simulink model "plant_model_us06_ev_V06"  (R2018a)
settings: Solver=ode3  StartTime=0.0  StopTime=sim_time  FixedStep=0.01  RelTol=1e-3
values from neighbouring files (symbols this model uses):
  A = 2.0    (= 2)    [plant_model_us06_ev_V06_m.m]
  Cd = 0.3    [plant_model_us06_ev_V06_m.m]
  FDR = 10    [plant_model_us06_ev_V06_m.m]
  g = 9.81    [plant_model_us06_ev_V06_m.m]
  initial_speed = 0    [plant_model_us06_ev_V06_m.m]
  M = 2000    [plant_model_us06_ev_V06_m.m]
  max_torque = 400    [plant_model_us06_ev_V06_m.m]
  Mr = 0.015    [plant_model_us06_ev_V06_m.m]
  p = 1.225    [plant_model_us06_ev_V06_m.m]
  power_kW = 100    [plant_model_us06_ev_V06_m.m]
  r = 0.35    [plant_model_us06_ev_V06_m.m]
  radiant_angle = 0    [plant_model_us06_ev_V06_m.m]
undefined symbols (not defined in the file or in its folder): magnitude
libraries: simulink x2
settings Model: Creator=satven  LastModifiedBy=satven

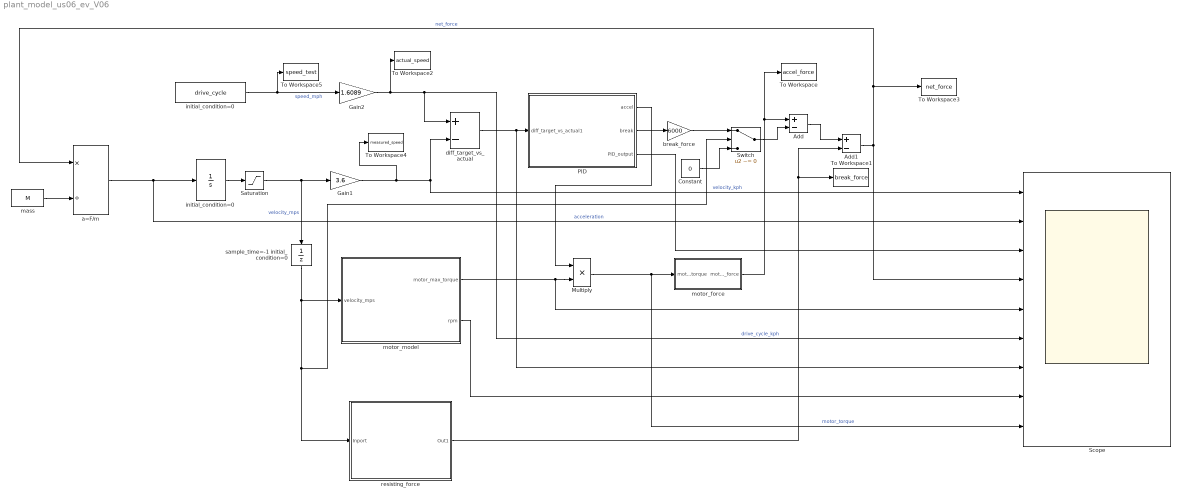
== system plant_model_us06_ev_V06 ==
  Add : Sum  Inputs=+-
  Add1 : Sum  Inputs=+-
  Constant : Constant  Value=0
  Gain1 : Gain  Gain=3.6
  Gain2 : Gain  Gain=1.6089
  Multiply : Product
  PID : Subsystem
  Saturation : Saturate  UpperLimit=inf  LowerLimit=0
  Scope : Scope  NumInputPorts=9
  Switch : Switch  Criteria=u2 ~= 0
  To Workspace : ToWorkspace  VariableName=accel_force  SaveFormat=Timeseries  SampleTime=-1
  To Workspace1 : ToWorkspace  VariableName=break_force  SaveFormat=Timeseries  SampleTime=-1
  To Workspace2 : ToWorkspace  VariableName=actual_speed  SaveFormat=Timeseries  SampleTime=-1
  To Workspace3 : ToWorkspace  VariableName=net_force  SaveFormat=Timeseries  SampleTime=-1
  To Workspace4 : ToWorkspace  VariableName=measured_speed  SaveFormat=Timeseries  SampleTime=-1
  To Workspace5 : ToWorkspace  VariableName=speed_test  SaveFormat=Timeseries  SampleTime=-1
  a=F/m : Product  Inputs=*/
  break_force : Gain  Gain=6000
  diff_target_vs_actual : Sum  Inputs=+-
  initial_condition=0 : Integrator  InitialCondition=initial_speed  LowerSaturationLimit=0
  "initial_condition=0 " : FromWorkspace  VariableName=drive_cycle  SampleTime=0.01
  mass : Constant  Value=M
  motor_force : Subsystem
  motor_model : Subsystem
  resisting_force : Subsystem
  "sample_time=-1 initial_condition=0 " : UnitDelay  SampleTime=-1
  wires:
  Gain1/1 -> To Workspace4/1, Scope/1, diff_target_vs_actual/2  "velocity_kph"
  diff_target_vs_actual/1 -> PID/1(diff_target_vs_actual1), Scope/7
  mass/1 -> a=F/m/2
  "sample_time=-1 initial_condition=0 "/1 -> motor_model/1(velocity_mps), Switch/2, resisting_force/1(Inport)
  a=F/m/1 -> initial_condition=0/1, Scope/2  "acceleration"
  Saturation/1 -> Gain1/1, "sample_time=-1 initial_condition=0 "/1  "velocity_mps"
  "initial_condition=0 "/1 -> Gain2/1, To Workspace5/1  "speed_mph"
  initial_condition=0/1 -> Saturation/1
  PID/3(PID_output) -> Scope/3
  Gain2/1 -> To Workspace2/1, diff_target_vs_actual/1, Scope/6  "drive_cycle_kph"
  Add/1 -> Add1/1
  PID/2(break) -> break_force/1
  motor_model/1(motor_max_torque) -> Scope/5, Multiply/2
  Add1/1 -> a=F/m/1, To Workspace3/1, Scope/4  "net_force"
  motor_model/2(rpm) -> Scope/8
  Multiply/1 -> Scope/9, motor_force/1(motor_torque)  "motor_torque"
  PID/1(accel) -> Multiply/1
  motor_force/1(motor_force) -> Add/1, To Workspace/1
  break_force/1 -> Switch/1
  Constant/1 -> Switch/3
  Switch/1 -> Add/2
  resisting_force/1(Out1) -> To Workspace1/1, Add1/2

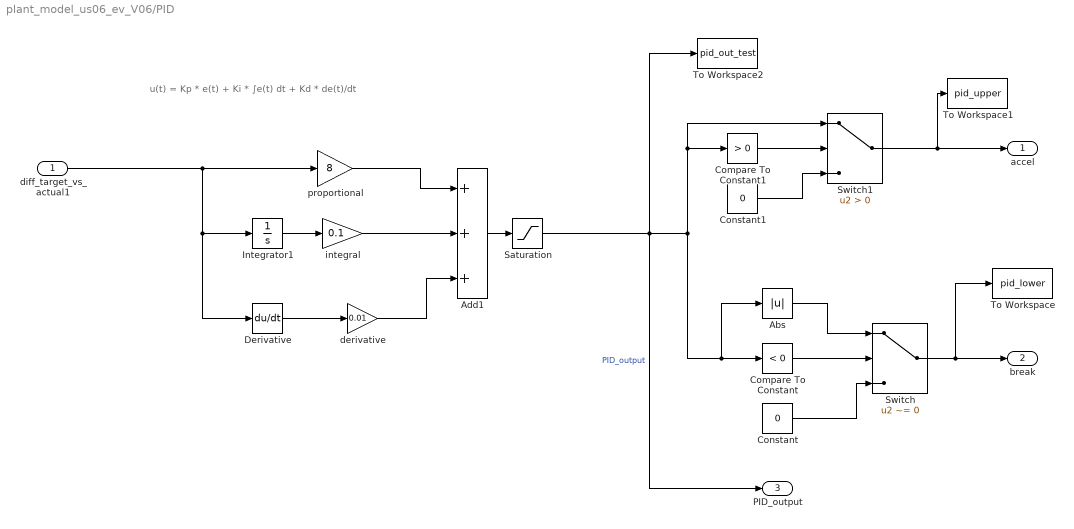
== system plant_model_us06_ev_V06/PID ==
  note: u(t) = Kp * e(t) + Ki * ∫e(t) dt + Kd * de(t)/dt
  diff_target_vs_actual1 : Inport
  Abs : Abs
  Add1 : Sum  Inputs=+++
  Compare To Constant : simulink/Logic and Bit Operations/Compare To Constant  relop=<  const=0  OutDataTypeStr=boolean
  Compare To Constant1 : simulink/Logic and Bit Operations/Compare To Constant  relop=>  const=0  OutDataTypeStr=boolean
  Constant : Constant  Value=0
  Constant1 : Constant  Value=0
  Derivative : Derivative
  Integrator1 : Integrator
  Saturation : Saturate  UpperLimit=1  LowerLimit=-1
  Switch : Switch  Criteria=u2 ~= 0
  Switch1 : Switch  Criteria=u2 > Threshold
  To Workspace : ToWorkspace  VariableName=pid_lower  SaveFormat=Timeseries  SampleTime=-1
  To Workspace1 : ToWorkspace  VariableName=pid_upper  SaveFormat=Timeseries  SampleTime=-1
  To Workspace2 : ToWorkspace  VariableName=pid_out_test  SaveFormat=Timeseries  SampleTime=-1
  "derivative " : Gain  Gain=0.01
  integral : Gain  Gain=0.1
  proportional : Gain  Gain=8
  accel : Outport
  break : Outport  Port=2
  PID_output : Outport  Port=3
  wires:
  proportional/1 -> Add1/1
  Derivative/1 -> "derivative "/1
  Integrator1/1 -> integral/1
  integral/1 -> Add1/2
  diff_target_vs_actual1/1 -> Derivative/1, Integrator1/1, proportional/1
  "derivative "/1 -> Add1/3
  Add1/1 -> Saturation/1
  Compare To Constant/1 -> Switch/2
  Compare To Constant1/1 -> Switch1/2
  Abs/1 -> Switch/1
  Constant/1 -> Switch/3
  Saturation/1 -> To Workspace2/1, PID_output/1, Abs/1, Compare To Constant/1, Switch1/1, Compare To Constant1/1  "PID_output"
  Switch/1 -> break/1, To Workspace/1
  Switch1/1 -> accel/1, To Workspace1/1
  Constant1/1 -> Switch1/3

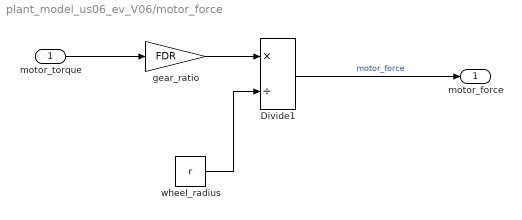
== system plant_model_us06_ev_V06/motor_force ==
  motor_torque : Inport
  Divide1 : Product  Inputs=*/
  gear_ratio : Gain  Gain=FDR
  wheel_radius : Constant  Value=r
  motor_force : Outport
  wires:
  motor_torque/1 -> gear_ratio/1
  wheel_radius/1 -> Divide1/2
  Divide1/1 -> motor_force/1  "motor_force"
  gear_ratio/1 -> Divide1/1

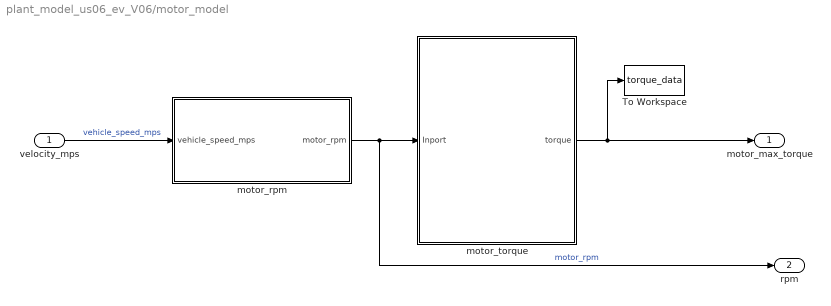
== system plant_model_us06_ev_V06/motor_model ==
  velocity_mps : Inport
  To Workspace : ToWorkspace  VariableName=torque_data  SaveFormat=Timeseries  SampleTime=-1
  motor_rpm : Subsystem
  motor_torque : Subsystem
  motor_max_torque : Outport
  rpm : Outport  Port=2
  wires:
  velocity_mps/1 -> motor_rpm/1(vehicle_speed_mps)  "vehicle_speed_mps"
  motor_torque/1(torque) -> To Workspace/1, motor_max_torque/1
  motor_rpm/1(motor_rpm) -> rpm/1, motor_torque/1(Inport)  "motor_rpm"

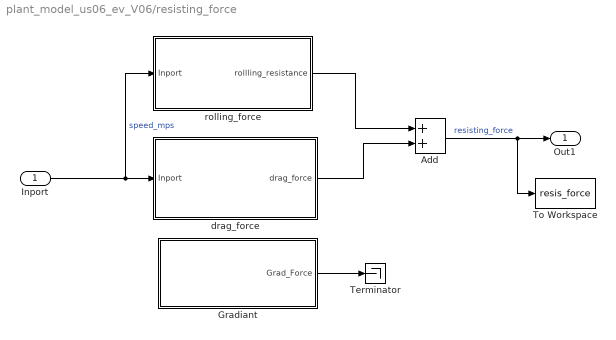
== system plant_model_us06_ev_V06/resisting_force ==
  Inport : Inport
  Add : Sum
  Gradiant : Subsystem
  Terminator : Terminator
  To Workspace : ToWorkspace  VariableName=resis_force  SaveFormat=Timeseries  SampleTime=-1
  drag_force : Subsystem
  rolling_force : Subsystem
  Out1 : Outport
  wires:
  drag_force/1(drag_force) -> Add/2
  Add/1 -> To Workspace/1, Out1/1  "resisting_force"
  rolling_force/1(rollling_resistance) -> Add/1
  Gradiant/1(Grad_Force) -> Terminator/1
  Inport/1 -> rolling_force/1(Inport), drag_force/1(Inport)  "speed_mps"

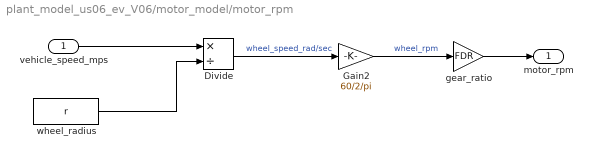
== system plant_model_us06_ev_V06/motor_model/motor_rpm ==
  vehicle_speed_mps : Inport
  Divide : Product  Inputs=*/
  Gain2 : Gain  Gain=60/2/pi
  gear_ratio : Gain  Gain=FDR
  wheel_radius : Constant  Value=r
  motor_rpm : Outport
  wires:
  wheel_radius/1 -> Divide/2
  Gain2/1 -> gear_ratio/1  "wheel_rpm"
  gear_ratio/1 -> motor_rpm/1
  Divide/1 -> Gain2/1  "wheel_speed_rad/sec"
  vehicle_speed_mps/1 -> Divide/1

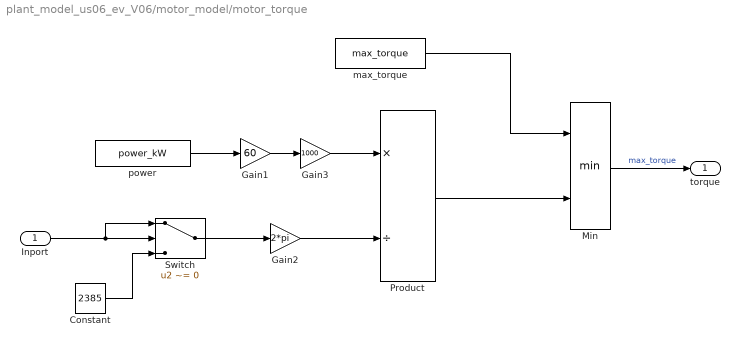
== system plant_model_us06_ev_V06/motor_model/motor_torque ==
  Inport : Inport
  Constant : Constant  Value=2385
  Gain1 : Gain  Gain=60
  Gain2 : Gain  Gain=2*pi
  Gain3 : Gain  Gain=1000
  Min : MinMax  Inputs=2
  Product : Product  Inputs=*/
  Switch : Switch  Criteria=u2 ~= 0
  max_torque : Constant  Value=max_torque
  power : Constant  Value=power_kW
  torque : Outport
  wires:
  power/1 -> Gain1/1
  Switch/1 -> Gain2/1
  Gain3/1 -> Product/1
  max_torque/1 -> Min/1
  Constant/1 -> Switch/3
  Gain2/1 -> Product/2
  Gain1/1 -> Gain3/1
  Product/1 -> Min/2
  Min/1 -> torque/1  "max_torque"
  Inport/1 -> Switch/1, Switch/2

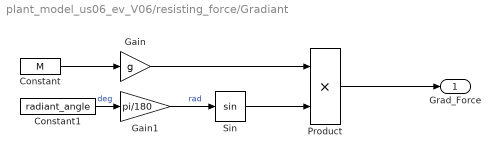
== system plant_model_us06_ev_V06/resisting_force/Gradiant ==
  Constant : Constant  Value=M
  Constant1 : Constant  Value=radiant_angle
  Gain : Gain  Gain=g
  Gain1 : Gain  Gain=pi/180
  Product : Product
  Sin : Trigonometry
  Grad_Force : Outport
  wires:
  Constant/1 -> Gain/1
  Product/1 -> Grad_Force/1
  Constant1/1 -> Gain1/1  "deg"
  Gain1/1 -> Sin/1  "rad"
  Gain/1 -> Product/1
  Sin/1 -> Product/2

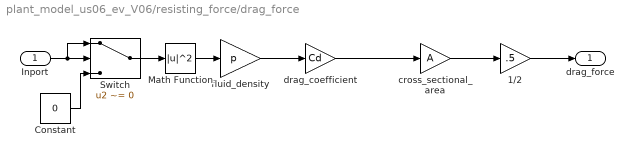
== system plant_model_us06_ev_V06/resisting_force/drag_force ==
  Inport : Inport
  1/2 : Gain  Gain=.5
  Constant : Constant  Value=0
  Math Function : Math  Operator=magnitude^2  OutputSignalType=real  SaturateOnIntegerOverflow=on
  Switch : Switch  Criteria=u2 ~= 0
  cross_sectional_area : Gain  Gain=A
  drag_coefficient : Gain  Gain=Cd
  fluid_density : Gain  Gain=p
  drag_force : Outport
  wires:
  Math Function/1 -> fluid_density/1
  fluid_density/1 -> drag_coefficient/1
  drag_coefficient/1 -> cross_sectional_area/1
  cross_sectional_area/1 -> 1/2/1
  1/2/1 -> drag_force/1
  Inport/1 -> Switch/2, Switch/1
  Switch/1 -> Math Function/1
  Constant/1 -> Switch/3

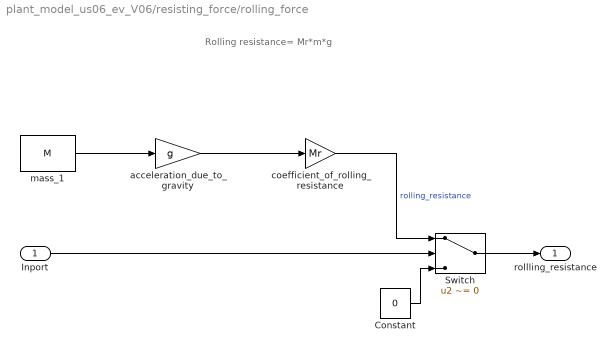
== system plant_model_us06_ev_V06/resisting_force/rolling_force ==
  note: Rolling resistance= Mr*m*g
  Inport : Inport
  Constant : Constant  Value=0
  Switch : Switch  Criteria=u2 ~= 0
  "acceleration_due_to_gravity " : Gain  Gain=g
  coefficient_of_rolling_resistance : Gain  Gain=Mr
  mass_1 : Constant  Value=M
  rollling_resistance : Outport
  wires:
  mass_1/1 -> "acceleration_due_to_gravity "/1
  "acceleration_due_to_gravity "/1 -> coefficient_of_rolling_resistance/1
  coefficient_of_rolling_resistance/1 -> Switch/1  "rolling_resistance"
  Constant/1 -> Switch/3
  Inport/1 -> Switch/2
  Switch/1 -> rollling_resistance/1
